simulink model "P2PHVDCMMC"  (R2024a)
settings: Solver=FixedStepDiscrete  StartTime=0.0  StopTime=10  RelTol=1e-3
PreLoadFcn:
  | % HVDCMMCInterconnectionParam
StartFcn:
  | tic
StopFcn:
  | toc
values from neighbouring files (symbols this model uses):
  C_PM = 1.758e-3    (= 0.001758)    [P2PHVDCMMCcode.m]    (also in SFu.mat)
  Cg = 50e-9    (= 5e-08)    [P2PHVDCMMCcode.m]    (also in SFu.mat)
  Fc = Fnom*3.37    (= 168.5)    [P2PHVDCMMCcode.m]    (also in SFu.mat)
  Fnom = 50    [P2PHVDCMMCcode.m]    (also in SFu.mat)
  HRM = 1    [SFu.mat]
  Ki_Ireg = 6    [P2PHVDCMMCcode.m]    (also in SFu.mat)
  Ki_Preg = 1.0    (= 1)    [P2PHVDCMMCcode.m]    (also in SFu.mat)
  Ki_Qreg = 1.0    (= 1)    [P2PHVDCMMCcode.m]    (also in SFu.mat)
  Ki_VDCreg = 100    [P2PHVDCMMCcode.m]    (also in SFu.mat)
  Kp_Ireg = 0.6    [P2PHVDCMMCcode.m]    (also in SFu.mat)
  Kp_Preg = 0.5/3    (= 0.166666666667)    [P2PHVDCMMCcode.m]    (also in SFu.mat)
  Kp_Qreg = 0.5/3    (= 0.166666666667)    [P2PHVDCMMCcode.m]    (also in SFu.mat)
  Kp_VDCreg = 4    [P2PHVDCMMCcode.m]    (also in SFu.mat)
  L_cable = 15e-3    (= 0.015)    [P2PHVDCMMCcode.m]    (also in SFu.mat)
  Larm = Larm_pu*(Zb_ac/(2*pi*Fnom))    [P2PHVDCMMCcode.m]    (also in SFu.mat = 0.0529455974536)
  Larm_pu = 0.15    [P2PHVDCMMCcode.m]    (also in SFu.mat)
  Lff = Larm_pu/2    (= 0.075)    [P2PHVDCMMCcode.m]    (also in SFu.mat)
  Limits_Ireg = [ 2.0  -2.0]    [P2PHVDCMMCcode.m]    (also in SFu.mat = [2 -2])
  Limits_Preg = [ 1.2, 0.8 ]    [P2PHVDCMMCcode.m]    (also in SFu.mat = [1.2 0.8])
  Limits_Qreg = [ 0.25, -0.25 ]    [P2PHVDCMMCcode.m]    (also in SFu.mat = [0.25 -0.25])
  Limits_VDCreg = [ 2.0  -2.0]    [P2PHVDCMMCcode.m]    (also in SFu.mat = [2 -2])
  Lxfo = 0.12    [P2PHVDCMMCcode.m]    (also in SFu.mat)
  N = 1    [P2PHVDCMMCcode.m]    (also in SFu.mat)
  Nb_PM = 36    [P2PHVDCMMCcode.m]    (also in SFu.mat)
  Pnom = 1000e6    (= 1000000000)    [P2PHVDCMMCcode.m]    (also in SFu.mat)
  R_cable = 0.5    [P2PHVDCMMCcode.m]    (also in SFu.mat)
  R_startup = 400    [P2PHVDCMMCcode.m]    (also in SFu.mat)
  Rarm = Rarm_pu*Zb_ac    [P2PHVDCMMCcode.m]    (also in SFu.mat = 0.1663335)
  Rff = Rarm_pu/2    (= 0.00075)    [P2PHVDCMMCcode.m]    (also in SFu.mat)
  Rg = 100    [P2PHVDCMMCcode.m]    (also in SFu.mat)
  Rxfo = 0.003    [P2PHVDCMMCcode.m]    (also in SFu.mat)
  S =     [SFu.mat]
  Slope_Qref = 0.5    [P2PHVDCMMCcode.m]    (also in SFu.mat)
  Slope_Vdc_ref = Vnom_dc/5    (= 128000)    [P2PHVDCMMCcode.m]    (also in SFu.mat)
  Tfault = 9999    [SFu.mat]
  Ts = Ts_Control    (= 4e-05)    [P2PHVDCMMCcode.m]    (also in SFu.mat)
  Ts_Control = 40e-6    (= 4e-05)    [P2PHVDCMMCcode.m]    (also in SFu.mat)
  Ts_dqn = 2e-5    (= 2e-05)    [P2PHVDCMMCcode.m]    (also in SFu.mat)
  Ts_Power = 20e-6    (= 2e-05)    [P2PHVDCMMCcode.m]    (also in SFu.mat)
  Vnom_dc = 640e3    (= 640000)    [P2PHVDCMMCcode.m]    (also in SFu.mat)
  Vnom_prim = 400e3    (= 400000)    [P2PHVDCMMCcode.m]    (also in SFu.mat)
  Vnom_sec = 333e3    (= 333000)    [P2PHVDCMMCcode.m]    (also in SFu.mat)
  Ws = 314.159265359    [SFu.mat]
undefined symbols (not defined in the file or in its folder): DiscIntNeverNeededParam, Discrete, DQN_Lib, gcbh, Int_DQNc_Mat, Mult_DQNc_Mat, Pcc, sps, sps_rtmsupport, spsMeanValueVariableFrequencyModel, spsPLL3phModel, SY3
libraries: simulink x38, spsControlledVoltageSourceLib x30, spsVoltageMeasurementLib x21, spsIdealSwitchLib x21, powerlib_extras x12, spsSecondOrderFilterLib x12, spsCurrentMeasurementLib x12, spsdq0toabcLib x9, spsMeanLib x8, spsMeanVariableFrequencyLib x8, spsabctodq0Lib x8, spsThreePhaseSeriesRLCBranchLib x7
(part 7 of 13)

== system P2PHVDCMMC/MMC AVG_Rec/Subsystem1/Circulating current suppression1/PI regulator with anti-windup D ==
  note: Anti-windup mechanism: Method of conditionnal integration
      |
      | The integration is suspended if saturation occurs and the
      | control error is of the same sign as the control signal.
      |
      | [1] L.Rundqwist, "Anti-Reset Windup for PID Controllers," Ph.D. Thesis TRFT-1033,
      | Departement of Automatic Control, Lund Institute of Technology, Lund, Sweeden, 1991.
  Error : Inport  SampleTime=Ts
  Compare To Zero : simulink/Logic and Bit Operations/Compare To Zero  relop=>  OutDataTypeStr=uint8  ZeroCross=off
  Compare To Zero1 : simulink/Logic and Bit Operations/Compare To Zero  relop=<  OutDataTypeStr=uint8  ZeroCross=off
  Constant : Constant  Value=0
  Constant1 : Constant  Value=UpperLimit
  Constant3 : Constant  Value=LowerLimit
  Discrete-Time Integrator : DiscreteIntegrator  IntegratorMethod=Integration: Trapezoidal  InitialCondition=Init  SampleTime=Ts  LimitOutput=on  UpperSaturationLimit=UpperLimit  LowerSaturationLimit=LowerLimit  ShowStatePort=on  ICPrevOutput=DiscIntNeverNeededParam  ICPrevScaledInput=DiscIntNeverNeededParam
  Kp4 : Gain  Gain=Kp  SaturateOnIntegerOverflow=on  SampleTime=Ts  OutDataTypeStr=Inherit: Same as input  ParamDataTypeStr=Inherit: Same as input
  Kp5 : Gain  Gain=Ki  SaturateOnIntegerOverflow=on  SampleTime=Ts  OutDataTypeStr=Inherit: Same as input  ParamDataTypeStr=Inherit: Same as input
  Logical Operator : Logic  AllPortsSameDT=off  OutDataTypeStr=boolean
  Logical Operator1 : Logic  AllPortsSameDT=off  OutDataTypeStr=boolean
  Logical Operator2 : Logic  Operator=OR  AllPortsSameDT=off  OutDataTypeStr=boolean
  Relational Operator : RelationalOperator  OutDataTypeStr=boolean  InputSameDT=off
  Relational Operator1 : RelationalOperator  Operator=<=  OutDataTypeStr=boolean  InputSameDT=off
  Saturation2 : Saturate  UpperLimit=UpperLimit  LowerLimit=LowerLimit  SampleTime=Ts
  Sum1 : Sum  InputSameDT=on  SaturateOnIntegerOverflow=on  SampleTime=Ts  OutDataTypeStr=Inherit: Same as first input
  Sum6 : Sum  InputSameDT=on  SaturateOnIntegerOverflow=on  SampleTime=Ts  OutDataTypeStr=Inherit: Same as first input
  Switch : Switch  Criteria=u2 > Threshold  SaturateOnIntegerOverflow=off  InputSameDT=off
  Zero-Order Hold : ZeroOrderHold  SampleTime=Ts
  Out : Outport  SampleTime=Ts  InitialOutput=0
  wires:
  Kp5/1 -> Switch/3
  Switch/1 -> Discrete-Time Integrator/1
  Saturation2/1 -> Out/1
  Discrete-Time Integrator/1 -> Sum6/2
  Kp4/1 -> Zero-Order Hold/1
  Sum6/1 -> Saturation2/1
  Error/1 -> Kp5/1, Kp4/1, Compare To Zero/1, Compare To Zero1/1
  Compare To Zero1/1 -> Logical Operator1/2  "Error_is_negative"
  Logical Operator1/1 -> Logical Operator2/2
  Logical Operator/1 -> Logical Operator2/1
  Compare To Zero/1 -> Logical Operator/2  "Error_is_positive"
  Constant3/1 -> Relational Operator1/2
  Constant1/1 -> Relational Operator/2
  Relational Operator1/1 -> Logical Operator1/1  "LowerLimit_Is_Reached"
  Relational Operator/1 -> Logical Operator/1  "UpperLimit_is_Reached"
  Logical Operator2/1 -> Switch/2
  Sum1/1 -> Relational Operator/1, Relational Operator1/1
  Discrete-Time Integrator/State -> Sum1/1
  Zero-Order Hold/1 -> Sum6/1, Sum1/2
  Constant/1 -> Switch/1

== system P2PHVDCMMC/MMC AVG_Rec/Subsystem1/Circulating current suppression1/PI regulator with anti-windup D1 ==
  note: Anti-windup mechanism: Method of conditionnal integration
      |
      | The integration is suspended if saturation occurs and the
      | control error is of the same sign as the control signal.
      |
      | [1] L.Rundqwist, "Anti-Reset Windup for PID Controllers," Ph.D. Thesis TRFT-1033,
      | Departement of Automatic Control, Lund Institute of Technology, Lund, Sweeden, 1991.
  Error : Inport  SampleTime=Ts
  Compare To Zero : simulink/Logic and Bit Operations/Compare To Zero  relop=>  OutDataTypeStr=uint8  ZeroCross=off
  Compare To Zero1 : simulink/Logic and Bit Operations/Compare To Zero  relop=<  OutDataTypeStr=uint8  ZeroCross=off
  Constant : Constant  Value=0
  Constant1 : Constant  Value=UpperLimit
  Constant3 : Constant  Value=LowerLimit
  Discrete-Time Integrator : DiscreteIntegrator  IntegratorMethod=Integration: Trapezoidal  InitialCondition=Init  SampleTime=Ts  LimitOutput=on  UpperSaturationLimit=UpperLimit  LowerSaturationLimit=LowerLimit  ShowStatePort=on  ICPrevOutput=DiscIntNeverNeededParam  ICPrevScaledInput=DiscIntNeverNeededParam
  Kp4 : Gain  Gain=Kp  SaturateOnIntegerOverflow=on  SampleTime=Ts  OutDataTypeStr=Inherit: Same as input  ParamDataTypeStr=Inherit: Same as input
  Kp5 : Gain  Gain=Ki  SaturateOnIntegerOverflow=on  SampleTime=Ts  OutDataTypeStr=Inherit: Same as input  ParamDataTypeStr=Inherit: Same as input
  Logical Operator : Logic  AllPortsSameDT=off  OutDataTypeStr=boolean
  Logical Operator1 : Logic  AllPortsSameDT=off  OutDataTypeStr=boolean
  Logical Operator2 : Logic  Operator=OR  AllPortsSameDT=off  OutDataTypeStr=boolean
  Relational Operator : RelationalOperator  OutDataTypeStr=boolean  InputSameDT=off
  Relational Operator1 : RelationalOperator  Operator=<=  OutDataTypeStr=boolean  InputSameDT=off
  Saturation2 : Saturate  UpperLimit=UpperLimit  LowerLimit=LowerLimit  SampleTime=Ts
  Sum1 : Sum  InputSameDT=on  SaturateOnIntegerOverflow=on  SampleTime=Ts  OutDataTypeStr=Inherit: Same as first input
  Sum6 : Sum  InputSameDT=on  SaturateOnIntegerOverflow=on  SampleTime=Ts  OutDataTypeStr=Inherit: Same as first input
  Switch : Switch  Criteria=u2 > Threshold  SaturateOnIntegerOverflow=off  InputSameDT=off
  Zero-Order Hold : ZeroOrderHold  SampleTime=Ts
  Out : Outport  SampleTime=Ts  InitialOutput=0
  wires:
  Constant/1 -> Switch/1
  Zero-Order Hold/1 -> Sum1/2, Sum6/1
  Discrete-Time Integrator/State -> Sum1/1
  Sum1/1 -> Relational Operator1/1, Relational Operator/1
  Logical Operator2/1 -> Switch/2
  Relational Operator/1 -> Logical Operator/1  "UpperLimit_is_Reached"
  Relational Operator1/1 -> Logical Operator1/1  "LowerLimit_Is_Reached"
  Constant1/1 -> Relational Operator/2
  Constant3/1 -> Relational Operator1/2
  Compare To Zero/1 -> Logical Operator/2  "Error_is_positive"
  Logical Operator/1 -> Logical Operator2/1
  Logical Operator1/1 -> Logical Operator2/2
  Compare To Zero1/1 -> Logical Operator1/2  "Error_is_negative"
  Error/1 -> Compare To Zero1/1, Compare To Zero/1, Kp4/1, Kp5/1
  Sum6/1 -> Saturation2/1
  Kp4/1 -> Zero-Order Hold/1
  Discrete-Time Integrator/1 -> Sum6/2
  Saturation2/1 -> Out/1
  Switch/1 -> Discrete-Time Integrator/1
  Kp5/1 -> Switch/3

== system P2PHVDCMMC/MMC AVG_Rec/Subsystem1/Subsystem/Subsystem ==
  g : Inport
  cb1 : spsIdealSwitchLib/Ideal Switch  Ron=0.001  Lon=0  IC=0  Rs=1e6  Cs=inf  Measurements=off
  cb2 : spsIdealSwitchLib/Ideal Switch  Ron=0.001  Lon=0  IC=0  Rs=1e6  Cs=inf  Measurements=off
  cb3 : spsIdealSwitchLib/Ideal Switch  Ron=0.001  Lon=0  IC=0  Rs=1e6  Cs=inf  Measurements=off
  1 : PMIOPort  Side=Left
  2 : PMIOPort  Port=2  Side=Left
  3 : PMIOPort  Port=3  Side=Left
  4 : PMIOPort  Port=4  Side=Right
  5 : PMIOPort  Port=5  Side=Right
  6 : PMIOPort  Port=6  Side=Right
  wires:
  g/1 -> cb3/1, cb2/1, cb1/1
  connections:
  cb3/RConn1 -- 6/RConn1
  cb3/LConn1 -- 3/RConn1
  cb2/RConn1 -- 5/RConn1
  cb1/LConn1 -- 1/RConn1
  cb1/RConn1 -- 4/RConn1
  cb2/LConn1 -- 2/RConn1

== system P2PHVDCMMC/MMC AVG_Rec/Subsystem1/Subsystem/Subsystem1 ==
  g : Inport
  cb4 : spsIdealSwitchLib/Ideal Switch  Ron=0.001  Lon=0  IC=0  Rs=1e6  Cs=inf  Measurements=off
  cb5 : spsIdealSwitchLib/Ideal Switch  Ron=0.001  Lon=0  IC=0  Rs=1e6  Cs=inf  Measurements=off
  cb6 : spsIdealSwitchLib/Ideal Switch  Ron=0.001  Lon=0  IC=0  Rs=1e6  Cs=inf  Measurements=off
  1 : PMIOPort  Side=Left
  2 : PMIOPort  Port=2  Side=Left
  3 : PMIOPort  Port=3  Side=Left
  4 : PMIOPort  Port=4  Side=Right
  5 : PMIOPort  Port=5  Side=Right
  6 : PMIOPort  Port=6  Side=Right
  wires:
  g/1 -> cb6/1, cb5/1, cb4/1
  connections:
  cb6/RConn1 -- 6/RConn1
  cb6/LConn1 -- 3/RConn1
  cb5/RConn1 -- 5/RConn1
  cb4/LConn1 -- 1/RConn1
  cb4/RConn1 -- 4/RConn1
  cb5/LConn1 -- 2/RConn1

== system P2PHVDCMMC/Subsystem4/ACinv/Circulating current suppression2/PI regulator with anti-windup D ==
  note: Anti-windup mechanism: Method of conditionnal integration
      |
      | The integration is suspended if saturation occurs and the
      | control error is of the same sign as the control signal.
      |
      | [1] L.Rundqwist, "Anti-Reset Windup for PID Controllers," Ph.D. Thesis TRFT-1033,
      | Departement of Automatic Control, Lund Institute of Technology, Lund, Sweeden, 1991.
  Error : Inport  SampleTime=Ts
  Compare To Zero : simulink/Logic and Bit Operations/Compare To Zero  relop=>  OutDataTypeStr=uint8  ZeroCross=off
  Compare To Zero1 : simulink/Logic and Bit Operations/Compare To Zero  relop=<  OutDataTypeStr=uint8  ZeroCross=off
  Constant : Constant  Value=0
  Constant1 : Constant  Value=UpperLimit
  Constant3 : Constant  Value=LowerLimit
  Discrete-Time Integrator : DiscreteIntegrator  IntegratorMethod=Integration: Trapezoidal  InitialCondition=Init  SampleTime=Ts  LimitOutput=on  UpperSaturationLimit=UpperLimit  LowerSaturationLimit=LowerLimit  ShowStatePort=on  ICPrevOutput=DiscIntNeverNeededParam  ICPrevScaledInput=DiscIntNeverNeededParam
  Kp4 : Gain  Gain=Kp  SaturateOnIntegerOverflow=on  SampleTime=Ts  OutDataTypeStr=Inherit: Same as input  ParamDataTypeStr=Inherit: Same as input
  Kp5 : Gain  Gain=Ki  SaturateOnIntegerOverflow=on  SampleTime=Ts  OutDataTypeStr=Inherit: Same as input  ParamDataTypeStr=Inherit: Same as input
  Logical Operator : Logic  AllPortsSameDT=off  OutDataTypeStr=boolean
  Logical Operator1 : Logic  AllPortsSameDT=off  OutDataTypeStr=boolean
  Logical Operator2 : Logic  Operator=OR  AllPortsSameDT=off  OutDataTypeStr=boolean
  Relational Operator : RelationalOperator  OutDataTypeStr=boolean  InputSameDT=off
  Relational Operator1 : RelationalOperator  Operator=<=  OutDataTypeStr=boolean  InputSameDT=off
  Saturation2 : Saturate  UpperLimit=UpperLimit  LowerLimit=LowerLimit  SampleTime=Ts
  Sum1 : Sum  InputSameDT=on  SaturateOnIntegerOverflow=on  SampleTime=Ts  OutDataTypeStr=Inherit: Same as first input
  Sum6 : Sum  InputSameDT=on  SaturateOnIntegerOverflow=on  SampleTime=Ts  OutDataTypeStr=Inherit: Same as first input
  Switch : Switch  Criteria=u2 > Threshold  SaturateOnIntegerOverflow=off  InputSameDT=off
  Zero-Order Hold : ZeroOrderHold  SampleTime=Ts
  Out : Outport  SampleTime=Ts  InitialOutput=0
  wires:
  Constant/1 -> Switch/1
  Zero-Order Hold/1 -> Sum1/2, Sum6/1
  Discrete-Time Integrator/State -> Sum1/1
  Sum1/1 -> Relational Operator1/1, Relational Operator/1
  Logical Operator2/1 -> Switch/2
  Relational Operator/1 -> Logical Operator/1  "UpperLimit_is_Reached"
  Relational Operator1/1 -> Logical Operator1/1  "LowerLimit_Is_Reached"
  Constant1/1 -> Relational Operator/2
  Constant3/1 -> Relational Operator1/2
  Compare To Zero/1 -> Logical Operator/2  "Error_is_positive"
  Logical Operator/1 -> Logical Operator2/1
  Logical Operator1/1 -> Logical Operator2/2
  Compare To Zero1/1 -> Logical Operator1/2  "Error_is_negative"
  Error/1 -> Compare To Zero1/1, Compare To Zero/1, Kp4/1, Kp5/1
  Sum6/1 -> Saturation2/1
  Kp4/1 -> Zero-Order Hold/1
  Discrete-Time Integrator/1 -> Sum6/2
  Saturation2/1 -> Out/1
  Switch/1 -> Discrete-Time Integrator/1
  Kp5/1 -> Switch/3

== system P2PHVDCMMC/Subsystem4/ACinv/Circulating current suppression2/PI regulator with anti-windup D1 ==
  note: Anti-windup mechanism: Method of conditionnal integration
      |
      | The integration is suspended if saturation occurs and the
      | control error is of the same sign as the control signal.
      |
      | [1] L.Rundqwist, "Anti-Reset Windup for PID Controllers," Ph.D. Thesis TRFT-1033,
      | Departement of Automatic Control, Lund Institute of Technology, Lund, Sweeden, 1991.
  Error : Inport  SampleTime=Ts
  Compare To Zero : simulink/Logic and Bit Operations/Compare To Zero  relop=>  OutDataTypeStr=uint8  ZeroCross=off
  Compare To Zero1 : simulink/Logic and Bit Operations/Compare To Zero  relop=<  OutDataTypeStr=uint8  ZeroCross=off
  Constant : Constant  Value=0
  Constant1 : Constant  Value=UpperLimit
  Constant3 : Constant  Value=LowerLimit
  Discrete-Time Integrator : DiscreteIntegrator  IntegratorMethod=Integration: Trapezoidal  InitialCondition=Init  SampleTime=Ts  LimitOutput=on  UpperSaturationLimit=UpperLimit  LowerSaturationLimit=LowerLimit  ShowStatePort=on  ICPrevOutput=DiscIntNeverNeededParam  ICPrevScaledInput=DiscIntNeverNeededParam
  Kp4 : Gain  Gain=Kp  SaturateOnIntegerOverflow=on  SampleTime=Ts  OutDataTypeStr=Inherit: Same as input  ParamDataTypeStr=Inherit: Same as input
  Kp5 : Gain  Gain=Ki  SaturateOnIntegerOverflow=on  SampleTime=Ts  OutDataTypeStr=Inherit: Same as input  ParamDataTypeStr=Inherit: Same as input
  Logical Operator : Logic  AllPortsSameDT=off  OutDataTypeStr=boolean
  Logical Operator1 : Logic  AllPortsSameDT=off  OutDataTypeStr=boolean
  Logical Operator2 : Logic  Operator=OR  AllPortsSameDT=off  OutDataTypeStr=boolean
  Relational Operator : RelationalOperator  OutDataTypeStr=boolean  InputSameDT=off
  Relational Operator1 : RelationalOperator  Operator=<=  OutDataTypeStr=boolean  InputSameDT=off
  Saturation2 : Saturate  UpperLimit=UpperLimit  LowerLimit=LowerLimit  SampleTime=Ts
  Sum1 : Sum  InputSameDT=on  SaturateOnIntegerOverflow=on  SampleTime=Ts  OutDataTypeStr=Inherit: Same as first input
  Sum6 : Sum  InputSameDT=on  SaturateOnIntegerOverflow=on  SampleTime=Ts  OutDataTypeStr=Inherit: Same as first input
  Switch : Switch  Criteria=u2 > Threshold  SaturateOnIntegerOverflow=off  InputSameDT=off
  Zero-Order Hold : ZeroOrderHold  SampleTime=Ts
  Out : Outport  SampleTime=Ts  InitialOutput=0
  wires:
  Kp5/1 -> Switch/3
  Switch/1 -> Discrete-Time Integrator/1
  Saturation2/1 -> Out/1
  Discrete-Time Integrator/1 -> Sum6/2
  Kp4/1 -> Zero-Order Hold/1
  Sum6/1 -> Saturation2/1
  Error/1 -> Kp5/1, Kp4/1, Compare To Zero/1, Compare To Zero1/1
  Compare To Zero1/1 -> Logical Operator1/2  "Error_is_negative"
  Logical Operator1/1 -> Logical Operator2/2
  Logical Operator/1 -> Logical Operator2/1
  Compare To Zero/1 -> Logical Operator/2  "Error_is_positive"
  Constant3/1 -> Relational Operator1/2
  Constant1/1 -> Relational Operator/2
  Relational Operator1/1 -> Logical Operator1/1  "LowerLimit_Is_Reached"
  Relational Operator/1 -> Logical Operator/1  "UpperLimit_is_Reached"
  Logical Operator2/1 -> Switch/2
  Sum1/1 -> Relational Operator/1, Relational Operator1/1
  Discrete-Time Integrator/State -> Sum1/1
  Zero-Order Hold/1 -> Sum6/1, Sum1/2
  Constant/1 -> Switch/1

== system P2PHVDCMMC/Subsystem4/ACrec/Circulating current suppression2/PI regulator with anti-windup D ==
  note: Anti-windup mechanism: Method of conditionnal integration
      |
      | The integration is suspended if saturation occurs and the
      | control error is of the same sign as the control signal.
      |
      | [1] L.Rundqwist, "Anti-Reset Windup for PID Controllers," Ph.D. Thesis TRFT-1033,
      | Departement of Automatic Control, Lund Institute of Technology, Lund, Sweeden, 1991.
  Error : Inport  SampleTime=Ts
  Compare To Zero : simulink/Logic and Bit Operations/Compare To Zero  relop=>  OutDataTypeStr=uint8  ZeroCross=off
  Compare To Zero1 : simulink/Logic and Bit Operations/Compare To Zero  relop=<  OutDataTypeStr=uint8  ZeroCross=off
  Constant : Constant  Value=0
  Constant1 : Constant  Value=UpperLimit
  Constant3 : Constant  Value=LowerLimit
  Discrete-Time Integrator : DiscreteIntegrator  IntegratorMethod=Integration: Trapezoidal  InitialCondition=Init  SampleTime=Ts  LimitOutput=on  UpperSaturationLimit=UpperLimit  LowerSaturationLimit=LowerLimit  ShowStatePort=on  ICPrevOutput=DiscIntNeverNeededParam  ICPrevScaledInput=DiscIntNeverNeededParam
  Kp4 : Gain  Gain=Kp  SaturateOnIntegerOverflow=on  SampleTime=Ts  OutDataTypeStr=Inherit: Same as input  ParamDataTypeStr=Inherit: Same as input
  Kp5 : Gain  Gain=Ki  SaturateOnIntegerOverflow=on  SampleTime=Ts  OutDataTypeStr=Inherit: Same as input  ParamDataTypeStr=Inherit: Same as input
  Logical Operator : Logic  AllPortsSameDT=off  OutDataTypeStr=boolean
  Logical Operator1 : Logic  AllPortsSameDT=off  OutDataTypeStr=boolean
  Logical Operator2 : Logic  Operator=OR  AllPortsSameDT=off  OutDataTypeStr=boolean
  Relational Operator : RelationalOperator  OutDataTypeStr=boolean  InputSameDT=off
  Relational Operator1 : RelationalOperator  Operator=<=  OutDataTypeStr=boolean  InputSameDT=off
  Saturation2 : Saturate  UpperLimit=UpperLimit  LowerLimit=LowerLimit  SampleTime=Ts
  Sum1 : Sum  InputSameDT=on  SaturateOnIntegerOverflow=on  SampleTime=Ts  OutDataTypeStr=Inherit: Same as first input
  Sum6 : Sum  InputSameDT=on  SaturateOnIntegerOverflow=on  SampleTime=Ts  OutDataTypeStr=Inherit: Same as first input
  Switch : Switch  Criteria=u2 > Threshold  SaturateOnIntegerOverflow=off  InputSameDT=off
  Zero-Order Hold : ZeroOrderHold  SampleTime=Ts
  Out : Outport  SampleTime=Ts  InitialOutput=0
  wires:
  Kp5/1 -> Switch/3
  Switch/1 -> Discrete-Time Integrator/1
  Saturation2/1 -> Out/1
  Discrete-Time Integrator/1 -> Sum6/2
  Kp4/1 -> Zero-Order Hold/1
  Sum6/1 -> Saturation2/1
  Error/1 -> Kp5/1, Kp4/1, Compare To Zero/1, Compare To Zero1/1
  Compare To Zero1/1 -> Logical Operator1/2  "Error_is_negative"
  Logical Operator1/1 -> Logical Operator2/2
  Logical Operator/1 -> Logical Operator2/1
  Compare To Zero/1 -> Logical Operator/2  "Error_is_positive"
  Constant3/1 -> Relational Operator1/2
  Constant1/1 -> Relational Operator/2
  Relational Operator1/1 -> Logical Operator1/1  "LowerLimit_Is_Reached"
  Relational Operator/1 -> Logical Operator/1  "UpperLimit_is_Reached"
  Logical Operator2/1 -> Switch/2
  Sum1/1 -> Relational Operator/1, Relational Operator1/1
  Discrete-Time Integrator/State -> Sum1/1
  Zero-Order Hold/1 -> Sum6/1, Sum1/2
  Constant/1 -> Switch/1

== system P2PHVDCMMC/Subsystem4/ACrec/Circulating current suppression2/PI regulator with anti-windup D1 ==
  note: Anti-windup mechanism: Method of conditionnal integration
      |
      | The integration is suspended if saturation occurs and the
      | control error is of the same sign as the control signal.
      |
      | [1] L.Rundqwist, "Anti-Reset Windup for PID Controllers," Ph.D. Thesis TRFT-1033,
      | Departement of Automatic Control, Lund Institute of Technology, Lund, Sweeden, 1991.
  Error : Inport  SampleTime=Ts
  Compare To Zero : simulink/Logic and Bit Operations/Compare To Zero  relop=>  OutDataTypeStr=uint8  ZeroCross=off
  Compare To Zero1 : simulink/Logic and Bit Operations/Compare To Zero  relop=<  OutDataTypeStr=uint8  ZeroCross=off
  Constant : Constant  Value=0
  Constant1 : Constant  Value=UpperLimit
  Constant3 : Constant  Value=LowerLimit
  Discrete-Time Integrator : DiscreteIntegrator  IntegratorMethod=Integration: Trapezoidal  InitialCondition=Init  SampleTime=Ts  LimitOutput=on  UpperSaturationLimit=UpperLimit  LowerSaturationLimit=LowerLimit  ShowStatePort=on  ICPrevOutput=DiscIntNeverNeededParam  ICPrevScaledInput=DiscIntNeverNeededParam
  Kp4 : Gain  Gain=Kp  SaturateOnIntegerOverflow=on  SampleTime=Ts  OutDataTypeStr=Inherit: Same as input  ParamDataTypeStr=Inherit: Same as input
  Kp5 : Gain  Gain=Ki  SaturateOnIntegerOverflow=on  SampleTime=Ts  OutDataTypeStr=Inherit: Same as input  ParamDataTypeStr=Inherit: Same as input
  Logical Operator : Logic  AllPortsSameDT=off  OutDataTypeStr=boolean
  Logical Operator1 : Logic  AllPortsSameDT=off  OutDataTypeStr=boolean
  Logical Operator2 : Logic  Operator=OR  AllPortsSameDT=off  OutDataTypeStr=boolean
  Relational Operator : RelationalOperator  OutDataTypeStr=boolean  InputSameDT=off
  Relational Operator1 : RelationalOperator  Operator=<=  OutDataTypeStr=boolean  InputSameDT=off
  Saturation2 : Saturate  UpperLimit=UpperLimit  LowerLimit=LowerLimit  SampleTime=Ts
  Sum1 : Sum  InputSameDT=on  SaturateOnIntegerOverflow=on  SampleTime=Ts  OutDataTypeStr=Inherit: Same as first input
  Sum6 : Sum  InputSameDT=on  SaturateOnIntegerOverflow=on  SampleTime=Ts  OutDataTypeStr=Inherit: Same as first input
  Switch : Switch  Criteria=u2 > Threshold  SaturateOnIntegerOverflow=off  InputSameDT=off
  Zero-Order Hold : ZeroOrderHold  SampleTime=Ts
  Out : Outport  SampleTime=Ts  InitialOutput=0
  wires:
  Constant/1 -> Switch/1
  Zero-Order Hold/1 -> Sum1/2, Sum6/1
  Discrete-Time Integrator/State -> Sum1/1
  Sum1/1 -> Relational Operator1/1, Relational Operator/1
  Logical Operator2/1 -> Switch/2
  Relational Operator/1 -> Logical Operator/1  "UpperLimit_is_Reached"
  Relational Operator1/1 -> Logical Operator1/1  "LowerLimit_Is_Reached"
  Constant1/1 -> Relational Operator/2
  Constant3/1 -> Relational Operator1/2
  Compare To Zero/1 -> Logical Operator/2  "Error_is_positive"
  Logical Operator/1 -> Logical Operator2/1
  Logical Operator1/1 -> Logical Operator2/2
  Compare To Zero1/1 -> Logical Operator1/2  "Error_is_negative"
  Error/1 -> Compare To Zero1/1, Compare To Zero/1, Kp4/1, Kp5/1
  Sum6/1 -> Saturation2/1
  Kp4/1 -> Zero-Order Hold/1
  Discrete-Time Integrator/1 -> Sum6/2
  Saturation2/1 -> Out/1
  Switch/1 -> Discrete-Time Integrator/1
  Kp5/1 -> Switch/3

== system P2PHVDCMMC/Control _DQn_inv/PLL, Measurements and Transformation1/PLL (3ph)/Model/Automatic Gain Control ==
  Freq : Inport
  Vdq : Inport  Port=2
  Enable : EnablePort  PropagateVarSize=During execution
  Math Function : Math  Operator=reciprocal  SignedPower=on
  Positive-Sequence (PLL-Driven) : Subsystem  AncestorBlock=|  DialogController=POWERSYS.PowerSysDialog  LoadFcn=sps_rtmsupport('LoadFcn', gcbh);  StartFcn=sps_rtmsupport('StartFcn', gcbh);  StopFcn=sps_rtmsupport('StopFcn', gcbh);  mask(Positive-Sequence (PLL-Driven)){Finit=sps.Finit, Fmin=sps.Fmin, InInit=[1 0], Ts=Ts}
      | sps_lib/Sensors and Measurements/Positive-Sequence
      | (PLL-Driven)
      mask prompts: Finit "Initial frequency (Hz):"; Fmin "Minimum frequency (Hz):"; InInit "Initial input (positive component)  [ Mag, Phase-relative-to-PLL (degrees) ]:"; Ts "Sample time:"
      mask help:
      | Compute the positive-sequence component of the input 3 signal over a running window of one cycle of fundamental frequency given by input 1. The signal can be a set of three balanced or unbalanced signals which may contain harmonics.
      | The reference frame required for the computation is given by the input 2.
      |
      | The two outputs return respectively the magnitude (same units as the input 3 signal) and phase (in degrees relative to the PLL phase) of the positive-sequence component of the abc input at the fundamental frequency.
      |
      | For the first cycle of simulation, the outputs are held constant to the values specified by the Initial input parameter. The Minimum frequency parameter is used to determine the buffer size of the Variable Transport Delay block used in the model.
      mask init:
      | [WantBlockChoice,Ts,sps] = powericon('PositiveSequencePLLDrivenInit',gcb,Finit,Fmin,InInit,Ts);
      settings: CopyFcn=sps_rtmsupport('CopyFcn', gcbh);  DeleteFcn=sps_rtmsupport('DeleteFcn', gcbh);  UndoDeleteFcn=sps_rtmsupport('UndoDeleteFcn', gcbh);  ModelCloseFcn=sps_rtmsupport('ModelCloseFcn', gcbh);  PreSaveFcn=sps_rtmsupport('PreSaveFcn', gcbh);  PostSaveFcn=sps_rtmsupport('PostSaveFcn', gcbh);  NameChangeFcn=sps_rtmsupport('NameChangeFcn', gcbh);  PreCopyFcn=sps_rtmsupport('PreCopyFcn', gcbh);  OpenFcn=sps_rtmsupport('OpenFcn', gcbh, []);  CloseFcn=sps_rtmsupport('CloseFcn', gcbh);  PreDeleteFcn=sps_rtmsupport('PreDeleteFcn', gcbh);
      settings: LibrarySourceBlock=|
      | sps_lib/Sensors and Measurements/Positive-Sequence
      | (PLL-Driven)
      mask Help: helpview(psbhelp);
      mask Display:
      | port_label('input',1,'Freq')
      | port_label('input',2,'wt')
      | port_label('input',3,'abc')
      | port_label('output',1,'|u|')
      | port_label('output',2,'\angleu', 'texmode', 'on')
  Saturation : Saturate  UpperLimit=inf  LowerLimit=eps
  Terminator1 : Terminator
  Gain : Outport  InitialOutput=[1]  VectorParamsAs1DForOutWhenUnconnected=off
  wires:
  Positive-Sequence (PLL-Driven)/1(Mag) -> Saturation/1
  Positive-Sequence (PLL-Driven)/2(Phase) -> Terminator1/1
  Math Function/1 -> Gain/1
  Vdq/1 -> Positive-Sequence (PLL-Driven)/2(dq)
  Freq/1 -> Positive-Sequence (PLL-Driven)/1(Freq)
  Saturation/1 -> Math Function/1

== system P2PHVDCMMC/Control _DQn_inv/PLL, Measurements and Transformation1/PLL (3ph)/Model/Discrete ==
  Err : Inport  SampleTime=Ts
  "Discrete Derivative " : DiscreteTransferFcn  Numerator="[ 1  -1 ]*Kd"  Denominator="[ TcD  Ts-TcD ]"  SampleTime=Ts
  Discrete-Time Integrator : DiscreteIntegrator  gainval=Ki  InitialCondition=Init  SampleTime=Ts  LimitOutput=on  UpperSaturationLimit=Par_Limits(1)  LowerSaturationLimit=Par_Limits(2)  ICPrevOutput=DiscIntNeverNeededParam  ICPrevScaledInput=DiscIntNeverNeededParam
  Kp4 : Gain  Gain=Kp  SaturateOnIntegerOverflow=on  SampleTime=Ts  OutDataTypeStr=Inherit: Same as input  ParamDataTypeStr=Inherit: Same as input
  Saturation1 : Saturate  UpperLimit=Par_Limits(1)  LowerLimit=Par_Limits(2)  SampleTime=Ts
  Sum6 : Sum  Inputs=+++  InputSameDT=on  SaturateOnIntegerOverflow=on  SampleTime=Ts  OutDataTypeStr=Inherit: Same as first input
  Out : Outport  SampleTime=Ts  InitialOutput=0  VectorParamsAs1DForOutWhenUnconnected=off
  wires:
  "Discrete Derivative "/1 -> Sum6/3
  Discrete-Time Integrator/1 -> Sum6/2
  Kp4/1 -> Sum6/1
  Sum6/1 -> Saturation1/1
  Err/1 -> "Discrete Derivative "/1, Kp4/1, Discrete-Time Integrator/1
  Saturation1/1 -> Out/1

== system P2PHVDCMMC/Control _DQn_inv/PLL, Measurements and Transformation1/PLL (3ph)/Model/Variable Frequency Mean value ==
  Freq : Inport  PortDimensions=1  SampleTime=Ts
  vq : Inport  Port=2  SampleTime=Ts
  Model : Subsystem  AncestorBlock=spsMeanValueVariableFrequencyModel/Discrete
  Mean : Outport  SampleTime=Ts  VectorParamsAs1DForOutWhenUnconnected=off
  wires:
  Model/1(Mean) -> Mean/1
  vq/1 -> Model/2(vq)
  Freq/1 -> Model/1(Freq)

== system P2PHVDCMMC/Control _DQn_inv/PLL, Measurements and Transformation1/PLL (3ph)2/Model/Automatic Gain Control ==
  Freq : Inport
  Vdq : Inport  Port=2
  Enable : EnablePort  PropagateVarSize=During execution
  Math Function : Math  Operator=reciprocal  SignedPower=on
  Positive-Sequence (PLL-Driven) : Subsystem  AncestorBlock=|  DialogController=POWERSYS.PowerSysDialog  LoadFcn=sps_rtmsupport('LoadFcn', gcbh);  StartFcn=sps_rtmsupport('StartFcn', gcbh);  StopFcn=sps_rtmsupport('StopFcn', gcbh);  mask(Positive-Sequence (PLL-Driven)){Finit=sps.Finit, Fmin=sps.Fmin, InInit=[1 0], Ts=Ts}
      | sps_lib/Sensors and Measurements/Positive-Sequence
      | (PLL-Driven)
      mask prompts: Finit "Initial frequency (Hz):"; Fmin "Minimum frequency (Hz):"; InInit "Initial input (positive component)  [ Mag, Phase-relative-to-PLL (degrees) ]:"; Ts "Sample time:"
      mask help:
      | Compute the positive-sequence component of the input 3 signal over a running window of one cycle of fundamental frequency given by input 1. The signal can be a set of three balanced or unbalanced signals which may contain harmonics.
      | The reference frame required for the computation is given by the input 2.
      |
      | The two outputs return respectively the magnitude (same units as the input 3 signal) and phase (in degrees relative to the PLL phase) of the positive-sequence component of the abc input at the fundamental frequency.
      |
      | For the first cycle of simulation, the outputs are held constant to the values specified by the Initial input parameter. The Minimum frequency parameter is used to determine the buffer size of the Variable Transport Delay block used in the model.
      mask init:
      | [WantBlockChoice,Ts,sps] = powericon('PositiveSequencePLLDrivenInit',gcb,Finit,Fmin,InInit,Ts);
      settings: CopyFcn=sps_rtmsupport('CopyFcn', gcbh);  DeleteFcn=sps_rtmsupport('DeleteFcn', gcbh);  UndoDeleteFcn=sps_rtmsupport('UndoDeleteFcn', gcbh);  ModelCloseFcn=sps_rtmsupport('ModelCloseFcn', gcbh);  PreSaveFcn=sps_rtmsupport('PreSaveFcn', gcbh);  PostSaveFcn=sps_rtmsupport('PostSaveFcn', gcbh);  NameChangeFcn=sps_rtmsupport('NameChangeFcn', gcbh);  PreCopyFcn=sps_rtmsupport('PreCopyFcn', gcbh);  OpenFcn=sps_rtmsupport('OpenFcn', gcbh, []);  CloseFcn=sps_rtmsupport('CloseFcn', gcbh);  PreDeleteFcn=sps_rtmsupport('PreDeleteFcn', gcbh);
      settings: LibrarySourceBlock=|
      | sps_lib/Sensors and Measurements/Positive-Sequence
      | (PLL-Driven)
      mask Help: helpview(psbhelp);
      mask Display:
      | port_label('input',1,'Freq')
      | port_label('input',2,'wt')
      | port_label('input',3,'abc')
      | port_label('output',1,'|u|')
      | port_label('output',2,'\angleu', 'texmode', 'on')
  Saturation : Saturate  UpperLimit=inf  LowerLimit=eps
  Terminator1 : Terminator
  Gain : Outport  InitialOutput=[1]  VectorParamsAs1DForOutWhenUnconnected=off
  wires:
  Positive-Sequence (PLL-Driven)/1(Mag) -> Saturation/1
  Positive-Sequence (PLL-Driven)/2(Phase) -> Terminator1/1
  Math Function/1 -> Gain/1
  Vdq/1 -> Positive-Sequence (PLL-Driven)/2(dq)
  Freq/1 -> Positive-Sequence (PLL-Driven)/1(Freq)
  Saturation/1 -> Math Function/1

== system P2PHVDCMMC/Control _DQn_inv/PLL, Measurements and Transformation1/PLL (3ph)2/Model/Discrete ==
  Err : Inport  SampleTime=Ts
  "Discrete Derivative " : DiscreteTransferFcn  Numerator="[ 1  -1 ]*Kd"  Denominator="[ TcD  Ts-TcD ]"  SampleTime=Ts
  Discrete-Time Integrator : DiscreteIntegrator  gainval=Ki  InitialCondition=Init  SampleTime=Ts  LimitOutput=on  UpperSaturationLimit=Par_Limits(1)  LowerSaturationLimit=Par_Limits(2)  ICPrevOutput=DiscIntNeverNeededParam  ICPrevScaledInput=DiscIntNeverNeededParam
  Kp4 : Gain  Gain=Kp  SaturateOnIntegerOverflow=on  SampleTime=Ts  OutDataTypeStr=Inherit: Same as input  ParamDataTypeStr=Inherit: Same as input
  Saturation1 : Saturate  UpperLimit=Par_Limits(1)  LowerLimit=Par_Limits(2)  SampleTime=Ts
  Sum6 : Sum  Inputs=+++  InputSameDT=on  SaturateOnIntegerOverflow=on  SampleTime=Ts  OutDataTypeStr=Inherit: Same as first input
  Out : Outport  SampleTime=Ts  InitialOutput=0  VectorParamsAs1DForOutWhenUnconnected=off
  wires:
  "Discrete Derivative "/1 -> Sum6/3
  Discrete-Time Integrator/1 -> Sum6/2
  Kp4/1 -> Sum6/1
  Sum6/1 -> Saturation1/1
  Err/1 -> "Discrete Derivative "/1, Kp4/1, Discrete-Time Integrator/1
  Saturation1/1 -> Out/1

== system P2PHVDCMMC/Control _DQn_inv/PLL, Measurements and Transformation1/PLL (3ph)2/Model/Variable Frequency Mean value ==
  Freq : Inport  PortDimensions=1  SampleTime=Ts
  vq : Inport  Port=2  SampleTime=Ts
  Model : Subsystem  AncestorBlock=spsMeanValueVariableFrequencyModel/Discrete
  Mean : Outport  SampleTime=Ts  VectorParamsAs1DForOutWhenUnconnected=off
  wires:
  Model/1(Mean) -> Mean/1
  vq/1 -> Model/2(vq)
  Freq/1 -> Model/1(Freq)

== system P2PHVDCMMC/Control _DQn_rec/PLL, Measurements and Transformation1/PLL (3ph)/Model/Automatic Gain Control ==
  Freq : Inport
  Vdq : Inport  Port=2
  Enable : EnablePort  PropagateVarSize=During execution
  Math Function : Math  Operator=reciprocal  SignedPower=on
  Positive-Sequence (PLL-Driven) : Subsystem  AncestorBlock=|  DialogController=POWERSYS.PowerSysDialog  LoadFcn=sps_rtmsupport('LoadFcn', gcbh);  StartFcn=sps_rtmsupport('StartFcn', gcbh);  StopFcn=sps_rtmsupport('StopFcn', gcbh);  mask(Positive-Sequence (PLL-Driven)){Finit=sps.Finit, Fmin=sps.Fmin, InInit=[1 0], Ts=Ts}
      | sps_lib/Sensors and Measurements/Positive-Sequence
      | (PLL-Driven)
      mask prompts: Finit "Initial frequency (Hz):"; Fmin "Minimum frequency (Hz):"; InInit "Initial input (positive component)  [ Mag, Phase-relative-to-PLL (degrees) ]:"; Ts "Sample time:"
      mask help:
      | Compute the positive-sequence component of the input 3 signal over a running window of one cycle of fundamental frequency given by input 1. The signal can be a set of three balanced or unbalanced signals which may contain harmonics.
      | The reference frame required for the computation is given by the input 2.
      |
      | The two outputs return respectively the magnitude (same units as the input 3 signal) and phase (in degrees relative to the PLL phase) of the positive-sequence component of the abc input at the fundamental frequency.
      |
      | For the first cycle of simulation, the outputs are held constant to the values specified by the Initial input parameter. The Minimum frequency parameter is used to determine the buffer size of the Variable Transport Delay block used in the model.
      mask init:
      | [WantBlockChoice,Ts,sps] = powericon('PositiveSequencePLLDrivenInit',gcb,Finit,Fmin,InInit,Ts);
      settings: CopyFcn=sps_rtmsupport('CopyFcn', gcbh);  DeleteFcn=sps_rtmsupport('DeleteFcn', gcbh);  UndoDeleteFcn=sps_rtmsupport('UndoDeleteFcn', gcbh);  ModelCloseFcn=sps_rtmsupport('ModelCloseFcn', gcbh);  PreSaveFcn=sps_rtmsupport('PreSaveFcn', gcbh);  PostSaveFcn=sps_rtmsupport('PostSaveFcn', gcbh);  NameChangeFcn=sps_rtmsupport('NameChangeFcn', gcbh);  PreCopyFcn=sps_rtmsupport('PreCopyFcn', gcbh);  OpenFcn=sps_rtmsupport('OpenFcn', gcbh, []);  CloseFcn=sps_rtmsupport('CloseFcn', gcbh);  PreDeleteFcn=sps_rtmsupport('PreDeleteFcn', gcbh);
      settings: LibrarySourceBlock=|
      | sps_lib/Sensors and Measurements/Positive-Sequence
      | (PLL-Driven)
      mask Help: helpview(psbhelp);
      mask Display:
      | port_label('input',1,'Freq')
      | port_label('input',2,'wt')
      | port_label('input',3,'abc')
      | port_label('output',1,'|u|')
      | port_label('output',2,'\angleu', 'texmode', 'on')
  Saturation : Saturate  UpperLimit=inf  LowerLimit=eps
  Terminator1 : Terminator
  Gain : Outport  InitialOutput=[1]  VectorParamsAs1DForOutWhenUnconnected=off
  wires:
  Positive-Sequence (PLL-Driven)/1(Mag) -> Saturation/1
  Positive-Sequence (PLL-Driven)/2(Phase) -> Terminator1/1
  Math Function/1 -> Gain/1
  Vdq/1 -> Positive-Sequence (PLL-Driven)/2(dq)
  Freq/1 -> Positive-Sequence (PLL-Driven)/1(Freq)
  Saturation/1 -> Math Function/1

== system P2PHVDCMMC/Control _DQn_rec/PLL, Measurements and Transformation1/PLL (3ph)/Model/Discrete ==
  Err : Inport  SampleTime=Ts
  "Discrete Derivative " : DiscreteTransferFcn  Numerator="[ 1  -1 ]*Kd"  Denominator="[ TcD  Ts-TcD ]"  SampleTime=Ts
  Discrete-Time Integrator : DiscreteIntegrator  gainval=Ki  InitialCondition=Init  SampleTime=Ts  LimitOutput=on  UpperSaturationLimit=Par_Limits(1)  LowerSaturationLimit=Par_Limits(2)  ICPrevOutput=DiscIntNeverNeededParam  ICPrevScaledInput=DiscIntNeverNeededParam
  Kp4 : Gain  Gain=Kp  SaturateOnIntegerOverflow=on  SampleTime=Ts  OutDataTypeStr=Inherit: Same as input  ParamDataTypeStr=Inherit: Same as input
  Saturation1 : Saturate  UpperLimit=Par_Limits(1)  LowerLimit=Par_Limits(2)  SampleTime=Ts
  Sum6 : Sum  Inputs=+++  InputSameDT=on  SaturateOnIntegerOverflow=on  SampleTime=Ts  OutDataTypeStr=Inherit: Same as first input
  Out : Outport  SampleTime=Ts  InitialOutput=0  VectorParamsAs1DForOutWhenUnconnected=off
  wires:
  "Discrete Derivative "/1 -> Sum6/3
  Discrete-Time Integrator/1 -> Sum6/2
  Kp4/1 -> Sum6/1
  Sum6/1 -> Saturation1/1
  Err/1 -> "Discrete Derivative "/1, Kp4/1, Discrete-Time Integrator/1
  Saturation1/1 -> Out/1

== system P2PHVDCMMC/Control _DQn_rec/PLL, Measurements and Transformation1/PLL (3ph)/Model/Variable Frequency Mean value ==
  Freq : Inport  PortDimensions=1  SampleTime=Ts
  vq : Inport  Port=2  SampleTime=Ts
  Model : Subsystem  AncestorBlock=spsMeanValueVariableFrequencyModel/Discrete
  Mean : Outport  SampleTime=Ts  VectorParamsAs1DForOutWhenUnconnected=off
  wires:
  Model/1(Mean) -> Mean/1
  vq/1 -> Model/2(vq)
  Freq/1 -> Model/1(Freq)

== system P2PHVDCMMC/Control _DQn_rec/PLL, Measurements and Transformation1/PLL (3ph)2/Model/Automatic Gain Control ==
  Freq : Inport
  Vdq : Inport  Port=2
  Enable : EnablePort  PropagateVarSize=During execution
  Math Function : Math  Operator=reciprocal  SignedPower=on
  Positive-Sequence (PLL-Driven) : Subsystem  AncestorBlock=|  DialogController=POWERSYS.PowerSysDialog  LoadFcn=sps_rtmsupport('LoadFcn', gcbh);  StartFcn=sps_rtmsupport('StartFcn', gcbh);  StopFcn=sps_rtmsupport('StopFcn', gcbh);  mask(Positive-Sequence (PLL-Driven)){Finit=sps.Finit, Fmin=sps.Fmin, InInit=[1 0], Ts=Ts}
      | sps_lib/Sensors and Measurements/Positive-Sequence
      | (PLL-Driven)
      mask prompts: Finit "Initial frequency (Hz):"; Fmin "Minimum frequency (Hz):"; InInit "Initial input (positive component)  [ Mag, Phase-relative-to-PLL (degrees) ]:"; Ts "Sample time:"
      mask help:
      | Compute the positive-sequence component of the input 3 signal over a running window of one cycle of fundamental frequency given by input 1. The signal can be a set of three balanced or unbalanced signals which may contain harmonics.
      | The reference frame required for the computation is given by the input 2.
      |
      | The two outputs return respectively the magnitude (same units as the input 3 signal) and phase (in degrees relative to the PLL phase) of the positive-sequence component of the abc input at the fundamental frequency.
      |
      | For the first cycle of simulation, the outputs are held constant to the values specified by the Initial input parameter. The Minimum frequency parameter is used to determine the buffer size of the Variable Transport Delay block used in the model.
      mask init:
      | [WantBlockChoice,Ts,sps] = powericon('PositiveSequencePLLDrivenInit',gcb,Finit,Fmin,InInit,Ts);
      settings: CopyFcn=sps_rtmsupport('CopyFcn', gcbh);  DeleteFcn=sps_rtmsupport('DeleteFcn', gcbh);  UndoDeleteFcn=sps_rtmsupport('UndoDeleteFcn', gcbh);  ModelCloseFcn=sps_rtmsupport('ModelCloseFcn', gcbh);  PreSaveFcn=sps_rtmsupport('PreSaveFcn', gcbh);  PostSaveFcn=sps_rtmsupport('PostSaveFcn', gcbh);  NameChangeFcn=sps_rtmsupport('NameChangeFcn', gcbh);  PreCopyFcn=sps_rtmsupport('PreCopyFcn', gcbh);  OpenFcn=sps_rtmsupport('OpenFcn', gcbh, []);  CloseFcn=sps_rtmsupport('CloseFcn', gcbh);  PreDeleteFcn=sps_rtmsupport('PreDeleteFcn', gcbh);
      settings: LibrarySourceBlock=|
      | sps_lib/Sensors and Measurements/Positive-Sequence
      | (PLL-Driven)
      mask Help: helpview(psbhelp);
      mask Display:
      | port_label('input',1,'Freq')
      | port_label('input',2,'wt')
      | port_label('input',3,'abc')
      | port_label('output',1,'|u|')
      | port_label('output',2,'\angleu', 'texmode', 'on')
  Saturation : Saturate  UpperLimit=inf  LowerLimit=eps
  Terminator1 : Terminator
  Gain : Outport  InitialOutput=[1]  VectorParamsAs1DForOutWhenUnconnected=off
  wires:
  Positive-Sequence (PLL-Driven)/1(Mag) -> Saturation/1
  Positive-Sequence (PLL-Driven)/2(Phase) -> Terminator1/1
  Math Function/1 -> Gain/1
  Vdq/1 -> Positive-Sequence (PLL-Driven)/2(dq)
  Freq/1 -> Positive-Sequence (PLL-Driven)/1(Freq)
  Saturation/1 -> Math Function/1

== system P2PHVDCMMC/Control _DQn_rec/PLL, Measurements and Transformation1/PLL (3ph)2/Model/Discrete ==
  Err : Inport  SampleTime=Ts
  "Discrete Derivative " : DiscreteTransferFcn  Numerator="[ 1  -1 ]*Kd"  Denominator="[ TcD  Ts-TcD ]"  SampleTime=Ts
  Discrete-Time Integrator : DiscreteIntegrator  gainval=Ki  InitialCondition=Init  SampleTime=Ts  LimitOutput=on  UpperSaturationLimit=Par_Limits(1)  LowerSaturationLimit=Par_Limits(2)  ICPrevOutput=DiscIntNeverNeededParam  ICPrevScaledInput=DiscIntNeverNeededParam
  Kp4 : Gain  Gain=Kp  SaturateOnIntegerOverflow=on  SampleTime=Ts  OutDataTypeStr=Inherit: Same as input  ParamDataTypeStr=Inherit: Same as input
  Saturation1 : Saturate  UpperLimit=Par_Limits(1)  LowerLimit=Par_Limits(2)  SampleTime=Ts
  Sum6 : Sum  Inputs=+++  InputSameDT=on  SaturateOnIntegerOverflow=on  SampleTime=Ts  OutDataTypeStr=Inherit: Same as first input
  Out : Outport  SampleTime=Ts  InitialOutput=0  VectorParamsAs1DForOutWhenUnconnected=off
  wires:
  "Discrete Derivative "/1 -> Sum6/3
  Discrete-Time Integrator/1 -> Sum6/2
  Kp4/1 -> Sum6/1
  Sum6/1 -> Saturation1/1
  Err/1 -> "Discrete Derivative "/1, Kp4/1, Discrete-Time Integrator/1
  Saturation1/1 -> Out/1

== system P2PHVDCMMC/Control _DQn_rec/PLL, Measurements and Transformation1/PLL (3ph)2/Model/Variable Frequency Mean value ==
  Freq : Inport  PortDimensions=1  SampleTime=Ts
  vq : Inport  Port=2  SampleTime=Ts
  Model : Subsystem  AncestorBlock=spsMeanValueVariableFrequencyModel/Discrete
  Mean : Outport  SampleTime=Ts  VectorParamsAs1DForOutWhenUnconnected=off
  wires:
  Model/1(Mean) -> Mean/1
  vq/1 -> Model/2(vq)
  Freq/1 -> Model/1(Freq)

== system P2PHVDCMMC/Control _DQn_inv/PLL, Measurements and Transformation1/PLL (3ph)/Model/Automatic Gain Control/Positive-Sequence (PLL-Driven) ==
  Freq : Inport  SampleTime=Ts
  dq : Inport  Port=2  SampleTime=Ts
  Complex to Magnitude-Angle : ComplexToMagnitudeAngle
  Mean (Variable Frequency)1 : spsMeanVariableFrequencyLib/Mean (Variable Frequency)  Finit=sps.Finit  Fmin=sps.Fmin  Vinit=sps.Real_Init  Ts=Ts
      settings: LibrarySourceBlock=|
      | sps_lib/Sensors and Measurements/Mean
      | (Variable Frequency)
  Mean (Variable Frequency)2 : spsMeanVariableFrequencyLib/Mean (Variable Frequency)  Finit=sps.Finit  Fmin=sps.Fmin  Vinit=sps.Imag_Init  Ts=Ts
      settings: LibrarySourceBlock=|
      | sps_lib/Sensors and Measurements/Mean
      | (Variable Frequency)
  Rad->Deg. : Gain  Gain=180/pi  SaturateOnIntegerOverflow=on  OutDataTypeStr=Inherit: Same as input  ParamDataTypeStr=Inherit: Same as input
  Real-Imag to Complex : RealImagToComplex
  Selector : Selector  InputPortWidth=2  IndexOptions=Index vector (dialog)  Indices=[1]  OutputSizes=1
  Selector1 : Selector  InputPortWidth=2  IndexOptions=Index vector (dialog)  Indices=[2]  OutputSizes=1
  Mag : Outport  SampleTime=Ts  VectorParamsAs1DForOutWhenUnconnected=off
  Phase : Outport  Port=2  SampleTime=Ts  VectorParamsAs1DForOutWhenUnconnected=off
  wires:
  Rad->Deg./1 -> Phase/1
  Mean (Variable Frequency)1/1 -> Real-Imag to Complex/1
  Freq/1 -> Mean (Variable Frequency)1/1, Mean (Variable Frequency)2/1
  Real-Imag to Complex/1 -> Complex to Magnitude-Angle/1
  Mean (Variable Frequency)2/1 -> Real-Imag to Complex/2
  Complex to Magnitude-Angle/1 -> Mag/1
  Complex to Magnitude-Angle/2 -> Rad->Deg./1
  dq/1 -> Selector/1, Selector1/1  "q"
  Selector/1 -> Mean (Variable Frequency)1/2  "d"
  Selector1/1 -> Mean (Variable Frequency)2/2  "q"

== system P2PHVDCMMC/Control _DQn_inv/PLL, Measurements and Transformation1/PLL (3ph)/Model/Variable Frequency Mean value/Model ==
  Freq : Inport  PortDimensions=1
  vq : Inport  Port=2
  Constant : Constant  Value=1/sps.Finit
  Correction subsystem : Subsystem
  Digital Clock : DigitalClock  SampleTime=Ts
  Discrete Variable Time Delay : spsDiscreteVariableTimeDelayLib/Discrete Variable Time Delay  MaxDelay=1/sps.Fmin+Ts  InitialValue=0  Ts=Ts  DFT=on
  Gain : Gain  Gain=Ts  SaturateOnIntegerOverflow=on  OutDataTypeStr=Inherit: Same as input  ParamDataTypeStr=Inherit: Same as input
  Integ4 : DiscreteIntegrator  IntegratorMethod=Integration: Trapezoidal  SampleTime=Ts  ICPrevOutput=DiscIntNeverNeededParam  ICPrevScaledInput=DiscIntNeverNeededParam
  Number of samples per cycle : Fcn  Expr=1/u[1]/Ts
  Product : Product  InputSameDT=on  SaturateOnIntegerOverflow=on  OutDataTypeStr=Inherit: Same as first input
  Relational Operator : RelationalOperator  OutDataTypeStr=boolean  SampleTime=Ts  InputSameDT=off
  Rounding Function : Rounding  Operator=ceil
  Sum5 : Sum  InputSameDT=on  SaturateOnIntegerOverflow=on  OutDataTypeStr=Inherit: Same as first input
  Sum7 : Sum  Inputs=-+  InputSameDT=on  SaturateOnIntegerOverflow=on  OutDataTypeStr=Inherit: Same as first input
  Switch : Switch  Threshold=0.5  SaturateOnIntegerOverflow=off
  To avoid division by zero : Saturate  UpperLimit=1e6  LowerLimit=eps
  Unit Delay1 : UnitDelay  InitialCondition=sps.Vinit  SampleTime=Ts  HasFrameUpgradeWarning=on
  Mean : Outport
  wires:
  Correction subsystem/1(Out) -> Sum5/2
  To avoid division by zero/1 -> Number of samples per cycle/1  "Freq"
  Switch/1 -> Mean/1, Unit Delay1/1
  Sum5/1 -> Switch/1
  Number of samples per cycle/1 -> Correction subsystem/1(N), Rounding Function/1
  Rounding Function/1 -> Correction subsystem/2(F), Gain/1
  Gain/1 -> Discrete Variable Time Delay/2  "Delay"
  Freq/1 -> To avoid division by zero/1, Product/2
  Integ4/1 -> Sum7/2, Discrete Variable Time Delay/1
  Sum7/1 -> Product/1
  Discrete Variable Time Delay/1 -> Sum7/1
  Product/1 -> Sum5/1  "Mean value"
  vq/1 -> Correction subsystem/3(In), Integ4/1
  Digital Clock/1 -> Relational Operator/1
  Unit Delay1/1 -> Switch/3
  Relational Operator/1 -> Switch/2
  Constant/1 -> Relational Operator/2

== system P2PHVDCMMC/Control _DQn_inv/PLL, Measurements and Transformation1/PLL (3ph)2/Model/Automatic Gain Control/Positive-Sequence (PLL-Driven) ==
  Freq : Inport  SampleTime=Ts
  dq : Inport  Port=2  SampleTime=Ts
  Complex to Magnitude-Angle : ComplexToMagnitudeAngle
  Mean (Variable Frequency)1 : spsMeanVariableFrequencyLib/Mean (Variable Frequency)  Finit=sps.Finit  Fmin=sps.Fmin  Vinit=sps.Real_Init  Ts=Ts
      settings: LibrarySourceBlock=|
      | sps_lib/Sensors and Measurements/Mean
      | (Variable Frequency)
  Mean (Variable Frequency)2 : spsMeanVariableFrequencyLib/Mean (Variable Frequency)  Finit=sps.Finit  Fmin=sps.Fmin  Vinit=sps.Imag_Init  Ts=Ts
      settings: LibrarySourceBlock=|
      | sps_lib/Sensors and Measurements/Mean
      | (Variable Frequency)
  Rad->Deg. : Gain  Gain=180/pi  SaturateOnIntegerOverflow=on  OutDataTypeStr=Inherit: Same as input  ParamDataTypeStr=Inherit: Same as input
  Real-Imag to Complex : RealImagToComplex
  Selector : Selector  InputPortWidth=2  IndexOptions=Index vector (dialog)  Indices=[1]  OutputSizes=1
  Selector1 : Selector  InputPortWidth=2  IndexOptions=Index vector (dialog)  Indices=[2]  OutputSizes=1
  Mag : Outport  SampleTime=Ts  VectorParamsAs1DForOutWhenUnconnected=off
  Phase : Outport  Port=2  SampleTime=Ts  VectorParamsAs1DForOutWhenUnconnected=off
  wires:
  Rad->Deg./1 -> Phase/1
  Mean (Variable Frequency)1/1 -> Real-Imag to Complex/1
  Freq/1 -> Mean (Variable Frequency)1/1, Mean (Variable Frequency)2/1
  Real-Imag to Complex/1 -> Complex to Magnitude-Angle/1
  Mean (Variable Frequency)2/1 -> Real-Imag to Complex/2
  Complex to Magnitude-Angle/1 -> Mag/1
  Complex to Magnitude-Angle/2 -> Rad->Deg./1
  dq/1 -> Selector/1, Selector1/1  "q"
  Selector/1 -> Mean (Variable Frequency)1/2  "d"
  Selector1/1 -> Mean (Variable Frequency)2/2  "q"
